simulink model "ep8_1_1"  (R2018a)
settings: Solver=FixedStepAuto  StartTime=0.0  StopTime=10.0  FixedStep=0.001  MaxStep=0.001  RelTol=1e-3
values from neighbouring files (symbols this model uses):
  dt = (tFinal-tStart)/50000    (= 0.0001)    [ep8_1.m]
  g = 9.8    [ep8_1.m]
  K = 0.8    [ep8_1.m]
settings Model: Creator=zheny  LastModifiedBy=zheny

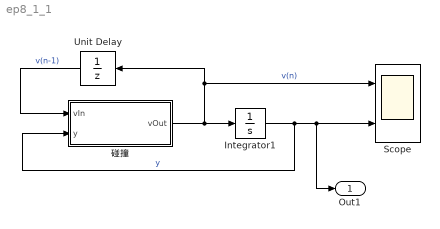
== system ep8_1_1 ==
  Integrator1 : Integrator  InitialCondition=1
  Scope : Scope  NumInputPorts=2
  Unit Delay : UnitDelay  SampleTime=dt
  碰撞 : Subsystem  mask(碰撞模型){K=K, g=g, dt=dt}
      mask init:
      | K = 0.8;
  Out1 : Outport
  wires:
  Integrator1/1 -> 碰撞/2(y), Out1/1, Scope/2  "y"
  碰撞/1(vOut) -> Scope/1, Unit Delay/1, Integrator1/1  "v(n)"
  Unit Delay/1 -> 碰撞/1(vIn)  "v(n-1)"

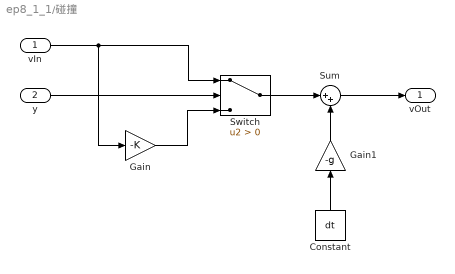
== system ep8_1_1/碰撞 ==
  vIn : Inport
  y : Inport  Port=2
  Constant : Constant  Value=dt
  Gain : Gain  Gain=-K
  Gain1 : Gain  Gain=-g
  Sum : Sum  Inputs=|++
  Switch : Switch  Criteria=u2 > Threshold
  vOut : Outport
  wires:
  vIn/1 -> Gain/1, Switch/1
  y/1 -> Switch/2
  Gain/1 -> Switch/3
  Switch/1 -> Sum/1
  Sum/1 -> vOut/1
  Constant/1 -> Gain1/1
  Gain1/1 -> Sum/2
